simulink model "block_schem"  (R2022a)
settings: Solver=VariableStepAuto  StartTime=0.0  StopTime=3e-5  RelTol=1e-6
values from neighbouring files (symbols this model uses):
  C1 = C1x    [MSE.m]
  C2 = C2x    [MSE.m]
  C3 = C3x    [MSE.m]
  L1 = L1x    [MSE.m]
  L2 = L2x    [MSE.m]
  L3 = L3x    [MSE.m]
  Rl = Rlx    (= 50)    [MSE.m]
  Rs = Rsx    (= 50)    [MSE.m]
libraries: slctrlblks x1
settings Model: Creator=vadym  LastModifiedBy=vadym

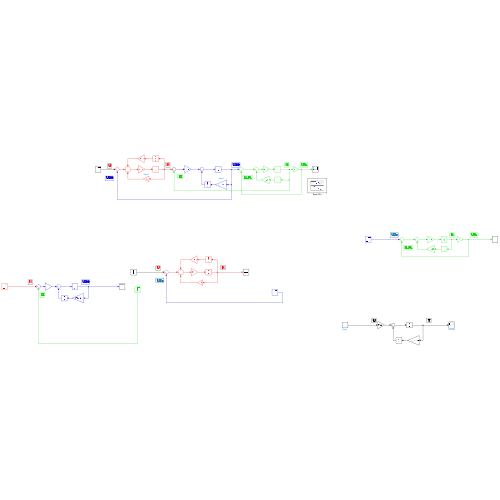
[thumbnail: Simulink's stored preview of the top-level diagram]
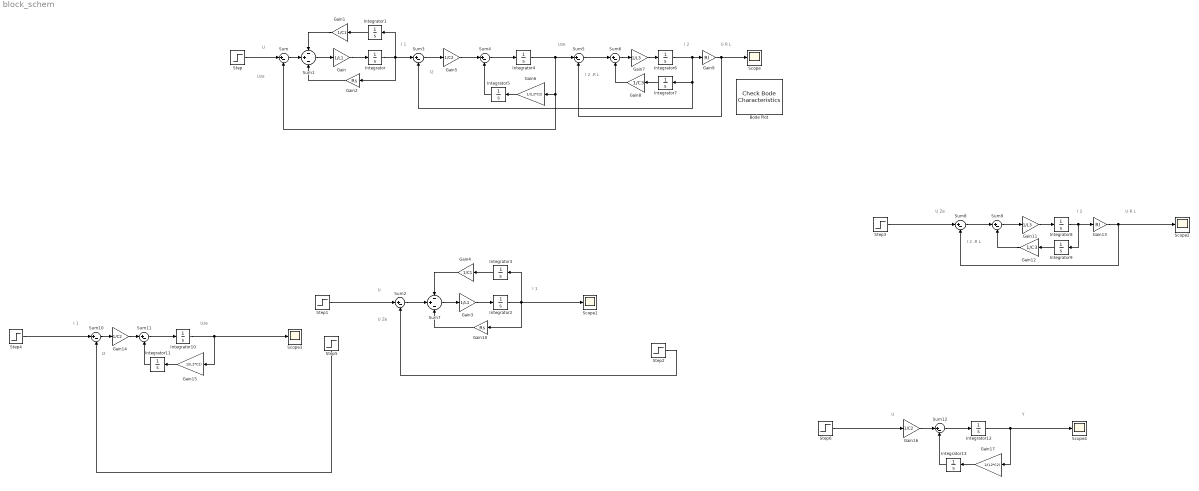
== system block_schem ==
  note: U R L
  note: U
  note: Uze
  note: I 1
  note: Uze
  note: I 2
  note: I 2 .R L
  note: U
  note: U Ze
  note: I 1
  note: I 2
  note: I 2 .R L
  note: U Ze
  note: U R L
  note: Uze
  note: I2
  note: I 1
  note: I2
  note: U
  note: Y
  Bode Plot : slctrlblks/Model Verification/Check Bode  Characteristics  InstantiateOnLoad=on  SaveOperatingPoints=off  LinearizationIOs={'/Step', 1, 'in', 'off', '';'/Gain9', 1, 'out', 'off', ''}  LinearizeAt=SnapshotTimes  SnapshotTimes=[0]  TriggerType=rising  SampleTime=auto  RateConversionMethod=zoh  PreWarpFreq=10  UseExactDelayModel=off  UseFullBlockNameLabels=off  UseBusSignalLabels=off  enabled=on  stopWhenAssertionFail=off  export=off  ViewDlgPos=[1 41 1536 748.8]  OpenViewOnLoad=off  LaunchViewOnOpen=on  FrequencyUnits=rad/s  MagnitudeUnits=dB  PhaseUnits=deg  TimeUnits=seconds  EnableUpperBound=off  UpperBoundFrequencies=[]  UpperBoundMagnitudes=[]  EnableLowerBound=off  LowerBoundFrequencies=[]  LowerBoundMagnitudes=[]
  Gain : Gain  Gain=1/L1
  Gain1 : Gain  Gain=1/C1
  Gain10 : Gain  Gain=Rs
  Gain11 : Gain  Gain=1/L3
  Gain12 : Gain  Gain=1/C3
  Gain13 : Gain  Gain=Rl
  Gain14 : Gain  Gain=1/C2
  Gain15 : Gain  Gain=1/(L2*C2)
  Gain16 : Gain  Gain=1/C2
  Gain17 : Gain  Gain=1/(L2*C2)
  Gain2 : Gain  Gain=Rs
  Gain3 : Gain  Gain=1/L1
  Gain4 : Gain  Gain=1/C1
  Gain5 : Gain  Gain=1/C2
  Gain6 : Gain  Gain=1/(L2*C2)
  Gain7 : Gain  Gain=1/L3
  Gain8 : Gain  Gain=1/C3
  Gain9 : Gain  Gain=Rl
  Integrator{,1..13} (14 alike) : Integrator
  Scope{,1..4} (5 alike) : Scope
  Step : Step  Time=0  SampleTime=0
  Step1 : Step  Time=0  SampleTime=0
  Step{2..6} (5 alike) : Step  SampleTime=0
  Sum{,2..6,8..12} (11 alike) : Sum  Inputs=|+-
  Sum1 : Sum  Inputs=-+-
  Sum7 : Sum  Inputs=-+-
  wires:
  Step/1 -> Sum/1
  Sum/1 -> Sum1/2
  Sum1/1 -> Gain/1
  Gain/1 -> Integrator/1
  Integrator/1 -> Sum3/1, Integrator1/1, Gain2/1
  Integrator1/1 -> Gain1/1
  Gain1/1 -> Sum1/1
  Sum3/1 -> Gain5/1
  Gain5/1 -> Sum4/1
  Sum4/1 -> Integrator4/1
  Integrator4/1 -> Sum/2, Gain6/1, Sum5/1
  Gain6/1 -> Integrator5/1
  Integrator5/1 -> Sum4/2
  Sum5/1 -> Sum6/1
  Sum6/1 -> Gain7/1
  Gain7/1 -> Integrator6/1
  Gain8/1 -> Sum6/2
  Integrator7/1 -> Gain8/1
  Integrator6/1 -> Gain9/1, Sum3/2, Integrator7/1
  Gain9/1 -> Scope/1, Sum5/2
  Gain2/1 -> Sum1/3
  Gain10/1 -> Sum7/3
  Integrator2/1 -> Scope1/1, Integrator3/1, Gain10/1
  Integrator3/1 -> Gain4/1
  Sum7/1 -> Gain3/1
  Sum2/1 -> Sum7/2
  Gain3/1 -> Integrator2/1
  Step1/1 -> Sum2/1
  Gain4/1 -> Sum7/1
  Step2/1 -> Sum2/2
  Gain12/1 -> Sum9/2
  Integrator8/1 -> Integrator9/1, Gain13/1
  Sum9/1 -> Gain11/1
  Gain13/1 -> Scope2/1, Sum8/2
  Integrator9/1 -> Gain12/1
  Gain11/1 -> Integrator8/1
  Sum8/1 -> Sum9/1
  Step3/1 -> Sum8/1
  Integrator10/1 -> Scope3/1, Gain15/1
  Sum10/1 -> Gain14/1
  Gain14/1 -> Sum11/1
  Sum11/1 -> Integrator10/1
  Gain15/1 -> Integrator11/1
  Step5/1 -> Sum10/2
  Integrator11/1 -> Sum11/2
  Step4/1 -> Sum10/1
  Integrator12/1 -> Scope4/1, Gain17/1
  Step6/1 -> Gain16/1
  Sum12/1 -> Integrator12/1
  Gain16/1 -> Sum12/1
  Gain17/1 -> Integrator13/1
  Integrator13/1 -> Sum12/2
